simulink model "robotarm"  (R2018b)
settings: Solver=FixedStepAuto  StartTime=0.0  StopTime=20  RelTol=1e-3  AbsTol=1e-6
undefined symbols (not defined in the file or in its folder): options
libraries: neural x132, simulink x2
(part 2 of 6)

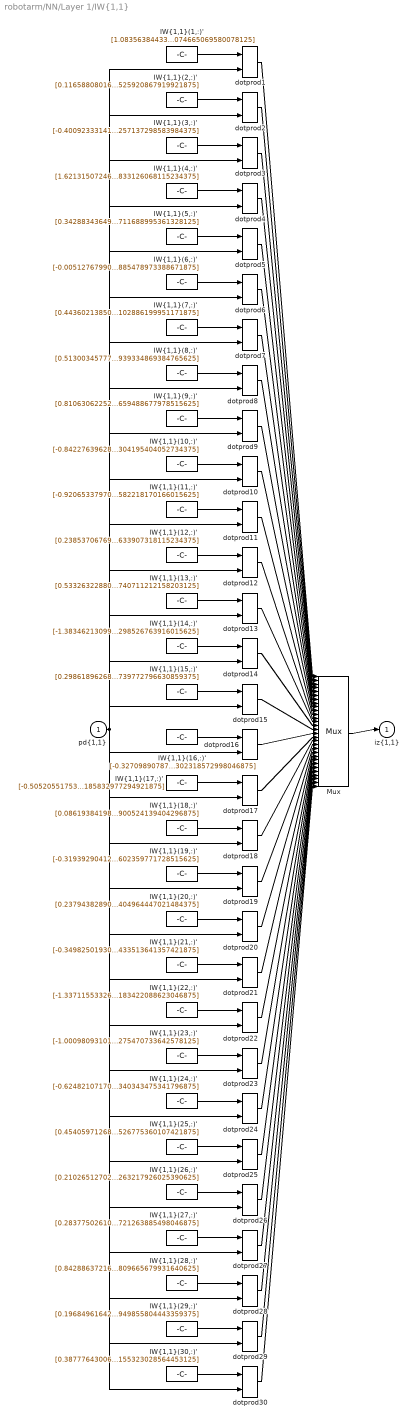
== system robotarm/NN/Layer 1/IW{1,1} ==
  "pd{1,1}" : Inport  PortDimensions=10
      mask Display: e = 0.06;c1 = [120 230 180]/255;c2 = ([120 230 180]+0)/(256+128);c3 = ([120 230 180]+128)/(256+128);patch([0 1 1 0],[0 0 1 1],c1);patch([0 1 1 1-e 1-e 0+e],[0 0 1 1-e 0+e 0+e],c2);patch([0 0 1 1-e 0+e 0+e],[0 1 1 1-e 1-e 0+e],c3);plot([0 1 1 0 0],[0 0 1 1 0]);
  "IW{1,1}(1,:)'" : Constant  Value=[1.083563844330424075224073021672666072845458984375;-0.419524106915114824989387898312998004257678985595703125;-0.94157120591915599572274686579476110637187957763671875;-0.01379674963687171039550261042450074455700814723968505859375;-0.58471965145644977379646434201276861131191253662109375;-0.280368088171196128133288993922178633511066436767578125;-0.31976801179407854380798426063847728073596954345703125;-0.52267253415010628270209736001561395823955535888671875;0.478910020528330815370310347134363837540149688720703125;0.1519211665722064730221774198071216233074665069580078125]
      mask Display: e = 0.06;c1 = [120 150 230]/255;c2 = ([120 150 230]+0)/383;c3 = ([120 150 230]+128)/383;patch([0 1 1 0],[0 0 1 1],c1);patch([0 1 1 1-e 1-e 0+e],[0 0 1 1-e 0+e 0+e],c2);patch([0 0 1 1-e 0+e 0+e],[0 1 1 1-e 1-e 0+e],c3);plot([0 1 1 0 0],[0 0 1 1 0]);disp('Weights');
  "IW{1,1}(10,:)'" : Constant  Value=[-0.842276396285047912471100062248297035694122314453125;-0.079177212965602150607224984923959709703922271728515625;0.61201067859849611618727749373647384345531463623046875;0.10430192382772003611979272363896598108112812042236328125;1.41024421573007874286531659890897572040557861328125;0.248495048171829047145564572929288260638713836669921875;-0.75706957483083592297390396197442896664142608642578125;0.472846624969997464393856034803320653736591339111328125;0.95744612924704741718784362092264927923679351806640625;1.4195525983288257432235468513681553304195404052734375]
      mask Display: e = 0.06;c1 = [120 150 230]/255;c2 = ([120 150 230]+0)/383;c3 = ([120 150 230]+128)/383;patch([0 1 1 0],[0 0 1 1],c1);patch([0 1 1 1-e 1-e 0+e],[0 0 1 1-e 0+e 0+e],c2);patch([0 0 1 1-e 0+e 0+e],[0 1 1 1-e 1-e 0+e],c3);plot([0 1 1 0 0],[0 0 1 1 0]);disp('Weights');
  "IW{1,1}(11,:)'" : Constant  Value=[-0.9206533797031231092233838353422470390796661376953125;1.000433613079543260226955680991522967815399169921875;-0.78174772750853949165872336379834450781345367431640625;0.9377401953158825964607103742309845983982086181640625;0.615533911757225826733019857783801853656768798828125;-1.301904266155556211259636256727389991283416748046875;-0.1439549990255313272058401707909069955348968505859375;-0.260988644890574217338752305295201949775218963623046875;-1.579813373534317832991291652433574199676513671875;0.3635611814509245309778862065286375582218170166015625]
      mask Display: e = 0.06;c1 = [120 150 230]/255;c2 = ([120 150 230]+0)/383;c3 = ([120 150 230]+128)/383;patch([0 1 1 0],[0 0 1 1],c1);patch([0 1 1 1-e 1-e 0+e],[0 0 1 1-e 0+e 0+e],c2);patch([0 0 1 1-e 0+e 0+e],[0 1 1 1-e 1-e 0+e],c3);plot([0 1 1 0 0],[0 0 1 1 0]);disp('Weights');
  "IW{1,1}(12,:)'" : Constant  Value=[0.2385370676987361993059977294251439161598682403564453125;-1.1182755603052239035122283894452266395092010498046875;0.30571718445612827697033253571134991943836212158203125;-0.12377321056275387978207191963520017452538013458251953125;-0.1540453467788618635569974912868929095566272735595703125;2.74495700415689203310876109753735363483428955078125;-2.15817502845816111545218518585897982120513916015625;0.12258293831009491048344983710194355808198451995849609375;0.435643584250738624685794775359681807458400726318359375;1.0191367826085675485359161029919050633907318115234375]
      mask Display: e = 0.06;c1 = [120 150 230]/255;c2 = ([120 150 230]+0)/383;c3 = ([120 150 230]+128)/383;patch([0 1 1 0],[0 0 1 1],c1);patch([0 1 1 1-e 1-e 0+e],[0 0 1 1-e 0+e 0+e],c2);patch([0 0 1 1-e 0+e 0+e],[0 1 1 1-e 1-e 0+e],c3);plot([0 1 1 0 0],[0 0 1 1 0]);disp('Weights');
  "IW{1,1}(13,:)'" : Constant  Value=[0.5332632288002676634874887895421124994754791259765625;-1.120563788042803654576573535450734198093414306640625;0.5760296974781053958025722749880515038967132568359375;0.1414568545696771317832229897248907946050167083740234375;-0.18376461551108647096697268352727405726909637451171875;0.748993908272824970850933823385275900363922119140625;-0.7624731059042806347036957959062419831752777099609375;0.1976752722123650551910856165704899467527866363525390625;0.07210207626949634296398272681472008116543292999267578125;0.5850282661990899857329395672422833740711212158203125]
      mask Display: e = 0.06;c1 = [120 150 230]/255;c2 = ([120 150 230]+0)/383;c3 = ([120 150 230]+128)/383;patch([0 1 1 0],[0 0 1 1],c1);patch([0 1 1 1-e 1-e 0+e],[0 0 1 1-e 0+e 0+e],c2);patch([0 0 1 1-e 0+e 0+e],[0 1 1 1-e 1-e 0+e],c3);plot([0 1 1 0 0],[0 0 1 1 0]);disp('Weights');
  "IW{1,1}(14,:)'" : Constant  Value=[-1.38346213099752279873655425035394728183746337890625;-0.6694901615044808185217561913304962217807769775390625;1.0052672642915541079133845414617098867893218994140625;-0.60839844430044476286667531894636340439319610595703125;1.978610543822657330537140296655707061290740966796875;0.08347416261820701788298748624583822675049304962158203125;-0.3532798783452408830640933956601656973361968994140625;-0.1049561498162090433794446653337217867374420166015625;-1.7363611870133974779406571542494930326938629150390625;0.2235057134043753335195248155287117697298526763916015625]
      mask Display: e = 0.06;c1 = [120 150 230]/255;c2 = ([120 150 230]+0)/383;c3 = ([120 150 230]+128)/383;patch([0 1 1 0],[0 0 1 1],c1);patch([0 1 1 1-e 1-e 0+e],[0 0 1 1-e 0+e 0+e],c2);patch([0 0 1 1-e 0+e 0+e],[0 1 1 1-e 1-e 0+e],c3);plot([0 1 1 0 0],[0 0 1 1 0]);disp('Weights');
  "IW{1,1}(15,:)'" : Constant  Value=[0.298618962681280020188268053971114568412303924560546875;-0.2574920415391714900721353842527605593204498291015625;0.286644932574378119571889556027599610388278961181640625;0.41670493839011901737734433481818996369838714599609375;0.9123539281340473650061539956368505954742431640625;-0.10092359044869168849256624298504902981221675872802734375;-1.363679620942679804329600301571190357208251953125;0.87390030526096407204050819927942939102649688720703125;0.1456549714138599682655694778077304363250732421875;0.58839728054712236993140095364651642739772796630859375]
      mask Display: e = 0.06;c1 = [120 150 230]/255;c2 = ([120 150 230]+0)/383;c3 = ([120 150 230]+128)/383;patch([0 1 1 0],[0 0 1 1],c1);patch([0 1 1 1-e 1-e 0+e],[0 0 1 1-e 0+e 0+e],c2);patch([0 0 1 1-e 0+e 0+e],[0 1 1 1-e 1-e 0+e],c3);plot([0 1 1 0 0],[0 0 1 1 0]);disp('Weights');
  "IW{1,1}(16,:)'" : Constant  Value=[-0.32709890787855167015862889456911943852901458740234375;-0.34977860185296594242032597321667708456516265869140625;0.159350112944072697107600333765731193125247955322265625;-0.4776914513121521821403803187422454357147216796875;0.28649800858607876730133057208149693906307220458984375;-1.6701621394718044744109874955029226839542388916015625;0.45311651717334289202199215651489794254302978515625;0.2452372552807220162929269235974061302840709686279296875;0.307275738364648998146577696388703770935535430908203125;-0.1802985558186971370986384499701671302318572998046875]
      mask Display: e = 0.06;c1 = [120 150 230]/255;c2 = ([120 150 230]+0)/383;c3 = ([120 150 230]+128)/383;patch([0 1 1 0],[0 0 1 1],c1);patch([0 1 1 1-e 1-e 0+e],[0 0 1 1-e 0+e 0+e],c2);patch([0 0 1 1-e 0+e 0+e],[0 1 1 1-e 1-e 0+e],c3);plot([0 1 1 0 0],[0 0 1 1 0]);disp('Weights');
  "IW{1,1}(17,:)'" : Constant  Value=[-0.505205517537357540192033411585725843906402587890625;0.73699201635039190971809830443817190825939178466796875;-0.91272025444561177831559461992583237588405609130859375;0.51464316420065514545711948812822811305522918701171875;-0.45956584150917467734842603022116236388683319091796875;0.266953627996282805145966676718671806156635284423828125;0.87997329801952528516295615190756507217884063720703125;0.56265541151544551379259928580722771584987640380859375;-0.81391511536075011878921259267372079193592071533203125;-0.17677379478027155368380363142932765185832977294921875]
      mask Display: e = 0.06;c1 = [120 150 230]/255;c2 = ([120 150 230]+0)/383;c3 = ([120 150 230]+128)/383;patch([0 1 1 0],[0 0 1 1],c1);patch([0 1 1 1-e 1-e 0+e],[0 0 1 1-e 0+e 0+e],c2);patch([0 0 1 1-e 0+e 0+e],[0 1 1 1-e 1-e 0+e],c3);plot([0 1 1 0 0],[0 0 1 1 0]);disp('Weights');
  "IW{1,1}(18,:)'" : Constant  Value=[0.08619384198746320169259860222155111841857433319091796875;0.229415038738241872096068618702702224254608154296875;0.422334408883638878773325586735154502093791961669921875;-0.0463857197077117422434611171411233954131603240966796875;-1.9378071193737458344230617512948811054229736328125;1.1617657080125656232638675646740011870861053466796875;0.72620292320079793402243240052484907209873199462890625;-0.266184247267512497092667445031111128628253936767578125;0.3750431508699769711512317371671088039875030517578125;0.12292905171981620415788682976199197582900524139404296875]
      mask Display: e = 0.06;c1 = [120 150 230]/255;c2 = ([120 150 230]+0)/383;c3 = ([120 150 230]+128)/383;patch([0 1 1 0],[0 0 1 1],c1);patch([0 1 1 1-e 1-e 0+e],[0 0 1 1-e 0+e 0+e],c2);patch([0 0 1 1-e 0+e 0+e],[0 1 1 1-e 1-e 0+e],c3);plot([0 1 1 0 0],[0 0 1 1 0]);disp('Weights');
  "IW{1,1}(19,:)'" : Constant  Value=[-0.319392904125261722914075335211236961185932159423828125;-1.11920722841916475687185084098018705844879150390625;1.2814339763144142469997177613549865782260894775390625;0.294714759578355245395187012036330997943878173828125;-0.127324947638250696169137654578662477433681488037109375;0.2780099290666580014175224278005771338939666748046875;-0.461406912688261894306407384647172875702381134033203125;0.946512221892773286668898435891605913639068603515625;-0.52604333433637762151846573033253662288188934326171875;1.12250699959288713358773748041130602359771728515625]
      mask Display: e = 0.06;c1 = [120 150 230]/255;c2 = ([120 150 230]+0)/383;c3 = ([120 150 230]+128)/383;patch([0 1 1 0],[0 0 1 1],c1);patch([0 1 1 1-e 1-e 0+e],[0 0 1 1-e 0+e 0+e],c2);patch([0 0 1 1-e 0+e 0+e],[0 1 1 1-e 1-e 0+e],c3);plot([0 1 1 0 0],[0 0 1 1 0]);disp('Weights');
  "IW{1,1}(2,:)'" : Constant  Value=[0.1165880801637612373955477096387767232954502105712890625;0.51480391570709194137833719651098363101482391357421875;0.85599582684588437775374814009410329163074493408203125;0.127689799126927516770280135460780002176761627197265625;-0.69251284680256031123235516133718192577362060546875;-0.77324080525538019248443788455915637314319610595703125;0.98812601958098100762839521848945878446102142333984375;-0.51915044520887076995308007099083624780178070068359375;0.35895177238562181454284427672973833978176116943359375;0.151165569358457652082705635621096007525920867919921875]
      mask Display: e = 0.06;c1 = [120 150 230]/255;c2 = ([120 150 230]+0)/383;c3 = ([120 150 230]+128)/383;patch([0 1 1 0],[0 0 1 1],c1);patch([0 1 1 1-e 1-e 0+e],[0 0 1 1-e 0+e 0+e],c2);patch([0 0 1 1-e 0+e 0+e],[0 1 1 1-e 1-e 0+e],c3);plot([0 1 1 0 0],[0 0 1 1 0]);disp('Weights');
  "IW{1,1}(20,:)'" : Constant  Value=[0.2379438289011180096554909368933294899761676788330078125;-1.3301846095986420426271479300339706242084503173828125;0.77044336265387458606568316099583171308040618896484375;-0.09547680704926130024201569312936044298112392425537109375;-2.715018010987653607202219063765369355678558349609375;2.072335550560776340489610447548329830169677734375;0.057260612174695142695401983701231074519455432891845703125;0.29725043610325474485733820984023623168468475341796875;-0.79005114949337118535055424217716790735721588134765625;-0.1293487886033327372015122591619729064404964447021484375]
      mask Display: e = 0.06;c1 = [120 150 230]/255;c2 = ([120 150 230]+0)/383;c3 = ([120 150 230]+128)/383;patch([0 1 1 0],[0 0 1 1],c1);patch([0 1 1 1-e 1-e 0+e],[0 0 1 1-e 0+e 0+e],c2);patch([0 0 1 1-e 0+e 0+e],[0 1 1 1-e 1-e 0+e],c3);plot([0 1 1 0 0],[0 0 1 1 0]);disp('Weights');
  "IW{1,1}(21,:)'" : Constant  Value=[-0.34982501930182452465345477321534417569637298583984375;0.451454660502078664041647471094620414078235626220703125;0.0176372183039427317396974359553496469743549823760986328125;0.5639563704868508775547297773300670087337493896484375;-0.61754695379530299970127771302941255271434783935546875;-1.1011264936744520337441599622252397239208221435546875;1.430952231708778388252767399535514414310455322265625;0.62703809529327825256217465721420012414455413818359375;0.89493822370913578279072453369735740125179290771484375;0.7420538838895331945622046987409703433513641357421875]
      mask Display: e = 0.06;c1 = [120 150 230]/255;c2 = ([120 150 230]+0)/383;c3 = ([120 150 230]+128)/383;patch([0 1 1 0],[0 0 1 1],c1);patch([0 1 1 1-e 1-e 0+e],[0 0 1 1-e 0+e 0+e],c2);patch([0 0 1 1-e 0+e 0+e],[0 1 1 1-e 1-e 0+e],c3);plot([0 1 1 0 0],[0 0 1 1 0]);disp('Weights');
  "IW{1,1}(22,:)'" : Constant  Value=[-1.3371155332655286773757552509778179228305816650390625;1.647611385498908731506162439472973346710205078125;0.7218372909033783368926151524647139012813568115234375;0.61517446653261964595316158010973595082759857177734375;0.4436209136289634979988250051974318921566009521484375;-0.618411794607119258415650620008818805217742919921875;0.03981089168389299881578580198038253001868724822998046875;0.204423240271942752155354128262843005359172821044921875;1.4694870831249475795488024232327006757259368896484375;0.34253618015753939385348303403588943183422088623046875]
      mask Display: e = 0.06;c1 = [120 150 230]/255;c2 = ([120 150 230]+0)/383;c3 = ([120 150 230]+128)/383;patch([0 1 1 0],[0 0 1 1],c1);patch([0 1 1 1-e 1-e 0+e],[0 0 1 1-e 0+e 0+e],c2);patch([0 0 1 1-e 0+e 0+e],[0 1 1 1-e 1-e 0+e],c3);plot([0 1 1 0 0],[0 0 1 1 0]);disp('Weights');
  "IW{1,1}(23,:)'" : Constant  Value=[-1.000980931013797370354723170748911798000335693359375;0.478833175182671821890068031279952265322208404541015625;0.94978064588756883068754177656956017017364501953125;1.1443594633221680911816520165302790701389312744140625;-0.11379400009978284102896139984295587055385112762451171875;0.74083642701004481789794908763724379241466522216796875;1.2769530613015283027067425791756249964237213134765625;-0.625360364122677925280413546715863049030303955078125;0.771054043074430150994658106355927884578704833984375;0.00902667251292374635263104920568366651423275470733642578125]
      mask Display: e = 0.06;c1 = [120 150 230]/255;c2 = ([120 150 230]+0)/383;c3 = ([120 150 230]+128)/383;patch([0 1 1 0],[0 0 1 1],c1);patch([0 1 1 1-e 1-e 0+e],[0 0 1 1-e 0+e 0+e],c2);patch([0 0 1 1-e 0+e 0+e],[0 1 1 1-e 1-e 0+e],c3);plot([0 1 1 0 0],[0 0 1 1 0]);disp('Weights');
  "IW{1,1}(24,:)'" : Constant  Value=[-0.6248210717015967308185508954920805990695953369140625;0.08457395706912758381879058333652210421860218048095703125;0.51798080722533257347350854615797288715839385986328125;-0.2401174058161140434375369068220607005059719085693359375;0.268766942934225816497217920186812989413738250732421875;-1.0091454203326735150625381720601581037044525146484375;0.3587305078967546467794136333395726978778839111328125;0.6470235736711653640185204494628123939037322998046875;-0.7765010235893623491421067228657193481922149658203125;-0.336555415051090267564148916790145449340343475341796875]
      mask Display: e = 0.06;c1 = [120 150 230]/255;c2 = ([120 150 230]+0)/383;c3 = ([120 150 230]+128)/383;patch([0 1 1 0],[0 0 1 1],c1);patch([0 1 1 1-e 1-e 0+e],[0 0 1 1-e 0+e 0+e],c2);patch([0 0 1 1-e 0+e 0+e],[0 1 1 1-e 1-e 0+e],c3);plot([0 1 1 0 0],[0 0 1 1 0]);disp('Weights');
  "IW{1,1}(25,:)'" : Constant  Value=[0.454059712686064653741624397298437543213367462158203125;-1.3517731457203157052759934231289662420749664306640625;0.1376707745836474316991626665185322053730487823486328125;-0.117666794937914265251066581186023540794849395751953125;0.1560771799800420300829983943913248367607593536376953125;-1.0269078294976130560911542488611303269863128662109375;-0.0027601815689167748073262753649714795756153762340545654296875;0.72699730352820690626458599581383168697357177734375;0.283288442579868571247203590246499516069889068603515625;1.308014024318274959313157523865811526775360107421875]
      mask Display: e = 0.06;c1 = [120 150 230]/255;c2 = ([120 150 230]+0)/383;c3 = ([120 150 230]+128)/383;patch([0 1 1 0],[0 0 1 1],c1);patch([0 1 1 1-e 1-e 0+e],[0 0 1 1-e 0+e 0+e],c2);patch([0 0 1 1-e 0+e 0+e],[0 1 1 1-e 1-e 0+e],c3);plot([0 1 1 0 0],[0 0 1 1 0]);disp('Weights');
  "IW{1,1}(26,:)'" : Constant  Value=[0.210265127027331522047148837373242713510990142822265625;-0.48581145213011378558576325303874909877777099609375;-0.123258874216255642775053047444089315831661224365234375;1.3525906749941525308855716502876020967960357666015625;-0.67024790288814617422730179896461777389049530029296875;-0.100694977273113772664459020234062336385250091552734375;-0.472021084205861474192289506390807218849658966064453125;-0.12293932717995796621845983054299722425639629364013671875;1.4301368055528242972940233812551014125347137451171875;-0.5388690494755474791332972017698921263217926025390625]
      mask Display: e = 0.06;c1 = [120 150 230]/255;c2 = ([120 150 230]+0)/383;c3 = ([120 150 230]+128)/383;patch([0 1 1 0],[0 0 1 1],c1);patch([0 1 1 1-e 1-e 0+e],[0 0 1 1-e 0+e 0+e],c2);patch([0 0 1 1-e 0+e 0+e],[0 1 1 1-e 1-e 0+e],c3);plot([0 1 1 0 0],[0 0 1 1 0]);disp('Weights');
  "IW{1,1}(27,:)'" : Constant  Value=[0.283775026102151828322206483790068887174129486083984375;-1.009030341954201492882248203386552631855010986328125;0.487583465416730976738080016730236820876598358154296875;-0.18846379806061719364151940681040287017822265625;-0.058983956930411328423158323630559607408940792083740234375;1.64386081481786394675737028592266142368316650390625;-0.40826383464646998078251272090710699558258056640625;0.033231970936722636522642204681687871925532817840576171875;-0.85776196289379547099684941713348962366580963134765625;-0.510846364679220510396362442406825721263885498046875]
      mask Display: e = 0.06;c1 = [120 150 230]/255;c2 = ([120 150 230]+0)/383;c3 = ([120 150 230]+128)/383;patch([0 1 1 0],[0 0 1 1],c1);patch([0 1 1 1-e 1-e 0+e],[0 0 1 1-e 0+e 0+e],c2);patch([0 0 1 1-e 0+e 0+e],[0 1 1 1-e 1-e 0+e],c3);plot([0 1 1 0 0],[0 0 1 1 0]);disp('Weights');
  "IW{1,1}(28,:)'" : Constant  Value=[0.84288637216753314884698511377791874110698699951171875;-0.413855342383396107575066480421810410916805267333984375;0.4049198819575854368935097227222286164760589599609375;-0.68308376935264780716039467733935452997684478759765625;-0.30854675245235763103579529342823661863803863525390625;-0.8917618698073483951560547211556695401668548583984375;-0.0897240545776623876772504218024550937116146087646484375;0.29103135192875873027418265337473712861537933349609375;0.5568927271626560315809228995931334793567657470703125;1.0573139604906318655963559649535454809665679931640625]
      mask Display: e = 0.06;c1 = [120 150 230]/255;c2 = ([120 150 230]+0)/383;c3 = ([120 150 230]+128)/383;patch([0 1 1 0],[0 0 1 1],c1);patch([0 1 1 1-e 1-e 0+e],[0 0 1 1-e 0+e 0+e],c2);patch([0 0 1 1-e 0+e 0+e],[0 1 1 1-e 1-e 0+e],c3);plot([0 1 1 0 0],[0 0 1 1 0]);disp('Weights');
  "IW{1,1}(29,:)'" : Constant  Value=[0.1968496164217669319729253629702725447714328765869140625;-1.4750248961380225676265354195493273437023162841796875;-0.0731711881804112673766127272756421007215976715087890625;-0.15866772515695803935642516080406494438648223876953125;0.25971984401405634468318339713732711970806121826171875;0.494830116170369038730569855033536441624164581298828125;-1.1275228062812632234823695398517884314060211181640625;0.387494119223098676396688233580789528787136077880859375;-0.260836540485615275830610926277586258947849273681640625;0.850286234828498521665096632204949855804443359375]
      mask Display: e = 0.06;c1 = [120 150 230]/255;c2 = ([120 150 230]+0)/383;c3 = ([120 150 230]+128)/383;patch([0 1 1 0],[0 0 1 1],c1);patch([0 1 1 1-e 1-e 0+e],[0 0 1 1-e 0+e 0+e],c2);patch([0 0 1 1-e 0+e 0+e],[0 1 1 1-e 1-e 0+e],c3);plot([0 1 1 0 0],[0 0 1 1 0]);disp('Weights');
  "IW{1,1}(3,:)'" : Constant  Value=[-0.400923331416590145170886216874350793659687042236328125;-0.1476879098288665925764462372171692550182342529296875;0.13125453123017549739159903765539638698101043701171875;0.04264655243906863291147857353280414827167987823486328125;0.72609917272249735464839659471181221306324005126953125;-1.075400786488810211949385120533406734466552734375;-0.0879519664267141842994846001602127216756343841552734375;0.11714601634093980975226401142208487726747989654541015625;1.68484348980962561626029128092341125011444091796875;0.145654699934613718337317322948365472257137298583984375]
      mask Display: e = 0.06;c1 = [120 150 230]/255;c2 = ([120 150 230]+0)/383;c3 = ([120 150 230]+128)/383;patch([0 1 1 0],[0 0 1 1],c1);patch([0 1 1 1-e 1-e 0+e],[0 0 1 1-e 0+e 0+e],c2);patch([0 0 1 1-e 0+e 0+e],[0 1 1 1-e 1-e 0+e],c3);plot([0 1 1 0 0],[0 0 1 1 0]);disp('Weights');
  "IW{1,1}(30,:)'" : Constant  Value=[0.387776430068318134214422343575279228389263153076171875;-0.0647149855580241017971587780266418121755123138427734375;-0.1699837310918328459052872858592309057712554931640625;-0.80075379385953004973686120138154365122318267822265625;-1.2626851263460927565773772585089318454265594482421875;0.011167974204610929545022912634522072039544582366943359375;-0.5182507885322260587912523988052271306514739990234375;1.2029977843526695746589894042699597775936126708984375;0.75153166640015722776979600894264876842498779296875;-0.50937516538142280086987057075020857155323028564453125]
      mask Display: e = 0.06;c1 = [120 150 230]/255;c2 = ([120 150 230]+0)/383;c3 = ([120 150 230]+128)/383;patch([0 1 1 0],[0 0 1 1],c1);patch([0 1 1 1-e 1-e 0+e],[0 0 1 1-e 0+e 0+e],c2);patch([0 0 1 1-e 0+e 0+e],[0 1 1 1-e 1-e 0+e],c3);plot([0 1 1 0 0],[0 0 1 1 0]);disp('Weights');
  "IW{1,1}(4,:)'" : Constant  Value=[1.6213150724644496136761517846025526523590087890625;-1.39679987700754093538080269354395568370819091796875;-0.332220191857820756897723413203493691980838775634765625;0.53809858749224026563950928903068415820598602294921875;0.63296520357793617517216944179381243884563446044921875;-0.59547763359107486191845737266703508794307708740234375;-0.1773979392923067111009771679164259694516658782958984375;-0.0418584878074302613182311461059725843369960784912109375;0.65839587112526920531507812484051100909709930419921875;-0.025669197067267078560259818686972721479833126068115234375]
      mask Display: e = 0.06;c1 = [120 150 230]/255;c2 = ([120 150 230]+0)/383;c3 = ([120 150 230]+128)/383;patch([0 1 1 0],[0 0 1 1],c1);patch([0 1 1 1-e 1-e 0+e],[0 0 1 1-e 0+e 0+e],c2);patch([0 0 1 1-e 0+e 0+e],[0 1 1 1-e 1-e 0+e],c3);plot([0 1 1 0 0],[0 0 1 1 0]);disp('Weights');
  "IW{1,1}(5,:)'" : Constant  Value=[0.342883436499595017910024807861191220581531524658203125;-1.041725722576007484576621209271252155303955078125;1.0054712358771265012791218396159820258617401123046875;-0.1703917873305470787048676584163331426680088043212890625;-1.1231709362679265229445491058868356049060821533203125;-0.8999364133153096023676198456087149679660797119140625;1.001279779505041656051389509229920804500579833984375;0.520364571732873759657422851887531578540802001953125;-0.90843751779553638669995052623562514781951904296875;-0.5052734573743038470894362035323865711688995361328125]
      mask Display: e = 0.06;c1 = [120 150 230]/255;c2 = ([120 150 230]+0)/383;c3 = ([120 150 230]+128)/383;patch([0 1 1 0],[0 0 1 1],c1);patch([0 1 1 1-e 1-e 0+e],[0 0 1 1-e 0+e 0+e],c2);patch([0 0 1 1-e 0+e 0+e],[0 1 1 1-e 1-e 0+e],c3);plot([0 1 1 0 0],[0 0 1 1 0]);disp('Weights');
  "IW{1,1}(6,:)'" : Constant  Value=[-0.005127679904386222599355082962802043766714632511138916015625;0.0253848319082346229880187138405744917690753936767578125;-0.62515248241674992168981361828627996146678924560546875;-0.1283637197299608845302287818412878550589084625244140625;-1.9671894012805564155854654018185101449489593505859375;1.0825371931026896987759755575098097324371337890625;0.035051283613600346666938634143662056885659694671630859375;0.749323223085553546951587122748605906963348388671875;-0.96344846650526727582786179482354782521724700927734375;0.357009315324879394903945240002940408885478973388671875]
      mask Display: e = 0.06;c1 = [120 150 230]/255;c2 = ([120 150 230]+0)/383;c3 = ([120 150 230]+128)/383;patch([0 1 1 0],[0 0 1 1],c1);patch([0 1 1 1-e 1-e 0+e],[0 0 1 1-e 0+e 0+e],c2);patch([0 0 1 1-e 0+e 0+e],[0 1 1 1-e 1-e 0+e],c3);plot([0 1 1 0 0],[0 0 1 1 0]);disp('Weights');
  "IW{1,1}(7,:)'" : Constant  Value=[0.443602138500584108893320944844163022935390472412109375;0.5897042425490841566215749480761587619781494140625;-0.07776107471227244882783224966260604560375213623046875;0.73813404077385735835292734918766655027866363525390625;-1.0677992091214718595182375793228857219219207763671875;1.0308052764952078117488554198644123971462249755859375;0.346772813933108547956862821592949330806732177734375;-0.15978460419619111565481262005050666630268096923828125;-0.577740532505497839110830682329833507537841796875;-1.103881593575507746862740532378666102886199951171875]
      mask Display: e = 0.06;c1 = [120 150 230]/255;c2 = ([120 150 230]+0)/383;c3 = ([120 150 230]+128)/383;patch([0 1 1 0],[0 0 1 1],c1);patch([0 1 1 1-e 1-e 0+e],[0 0 1 1-e 0+e 0+e],c2);patch([0 0 1 1-e 0+e 0+e],[0 1 1 1-e 1-e 0+e],c3);plot([0 1 1 0 0],[0 0 1 1 0]);disp('Weights');
  "IW{1,1}(8,:)'" : Constant  Value=[0.5130034577743221024803688123938627541065216064453125;-1.36132327419380683153349309577606618404388427734375;-0.184786816108494955646079915823065675795078277587890625;0.57684124394947866587557427919819019734859466552734375;-0.80847892494082407299771375619457103312015533447265625;0.13647065469038854867989130070782266557216644287109375;-0.69725806686932312317139803781174123287200927734375;-0.49791543974283591911245139272068627178668975830078125;0.5568004775091164315625746894511394202709197998046875;-0.56237914196716209946913522799150086939334869384765625]
      mask Display: e = 0.06;c1 = [120 150 230]/255;c2 = ([120 150 230]+0)/383;c3 = ([120 150 230]+128)/383;patch([0 1 1 0],[0 0 1 1],c1);patch([0 1 1 1-e 1-e 0+e],[0 0 1 1-e 0+e 0+e],c2);patch([0 0 1 1-e 0+e 0+e],[0 1 1 1-e 1-e 0+e],c3);plot([0 1 1 0 0],[0 0 1 1 0]);disp('Weights');
  "IW{1,1}(9,:)'" : Constant  Value=[0.810630622529874056425569506245665252208709716796875;0.13529562971586173159010968447546474635601043701171875;-0.08447588975580629100381457874391344375908374786376953125;0.173504432054140289576338318511261604726314544677734375;-1.2880709604838729287479281993000768125057220458984375;-1.4583641511193936590728981173015199601650238037109375;2.08180199668271370683214627206325531005859375;0.6387697649847867698014169945963658392429351806640625;-0.39397763097241222940425586784840561449527740478515625;-0.05706823956178132262184732326204539276659488677978515625]
      mask Display: e = 0.06;c1 = [120 150 230]/255;c2 = ([120 150 230]+0)/383;c3 = ([120 150 230]+128)/383;patch([0 1 1 0],[0 0 1 1],c1);patch([0 1 1 1-e 1-e 0+e],[0 0 1 1-e 0+e 0+e],c2);patch([0 0 1 1-e 0+e 0+e],[0 1 1 1-e 1-e 0+e],c3);plot([0 1 1 0 0],[0 0 1 1 0]);disp('Weights');
  Mux : Mux  Inputs=30
      mask Display: e = 0.06;c1 = [120 150 230]/255;c2 = ([120 150 230]+0)/383;c3 = ([120 150 230]+128)/383;patch([0 1 1 0],[0 0 1 1],c1);patch([0 1 1 1-e 1-e 0+e],[0 0 1 1-e 0+e 0+e],c2);patch([0 0 1 1-e 0+e 0+e],[0 1 1 1-e 1-e 0+e],c3);plot([0 1 1 0 0],[0 0 1 1 0]);disp('Mux');
  dotprod{1..30} (30 alike) : neural/Weight Functions/dotprod
  "iz{1,1}" : Outport
      mask Display: e = 0.06;c1 = [120 230 180]/255;c2 = ([120 230 180]+0)/(256+128);c3 = ([120 230 180]+128)/(256+128);patch([0 1 1 0],[0 0 1 1],c1);patch([0 1 1 1-e 1-e 0+e],[0 0 1 1-e 0+e 0+e],c2);patch([0 0 1 1-e 0+e 0+e],[0 1 1 1-e 1-e 0+e],c3);plot([0 1 1 0 0],[0 0 1 1 0]);
  wires:
  "IW{1,1}(1,:)'"/1 -> dotprod1/1
  "pd{1,1}"/1 -> dotprod1/2, dotprod2/2, dotprod3/2, dotprod4/2, dotprod5/2, dotprod6/2, dotprod7/2, dotprod8/2, dotprod9/2, dotprod10/2, dotprod11/2, dotprod12/2, dotprod13/2, dotprod14/2, dotprod15/2, dotprod16/2, dotprod17/2, dotprod18/2, dotprod19/2, dotprod20/2, dotprod21/2, dotprod22/2, dotprod23/2, dotprod24/2, dotprod25/2, dotprod26/2, dotprod27/2, dotprod28/2, dotprod29/2, dotprod30/2
  dotprod1/1 -> Mux/1
  "IW{1,1}(2,:)'"/1 -> dotprod2/1
  dotprod2/1 -> Mux/2
  "IW{1,1}(3,:)'"/1 -> dotprod3/1
  dotprod3/1 -> Mux/3
  "IW{1,1}(4,:)'"/1 -> dotprod4/1
  dotprod4/1 -> Mux/4
  "IW{1,1}(5,:)'"/1 -> dotprod5/1
  dotprod5/1 -> Mux/5
  "IW{1,1}(6,:)'"/1 -> dotprod6/1
  dotprod6/1 -> Mux/6
  "IW{1,1}(7,:)'"/1 -> dotprod7/1
  dotprod7/1 -> Mux/7
  "IW{1,1}(8,:)'"/1 -> dotprod8/1
  dotprod8/1 -> Mux/8
  "IW{1,1}(9,:)'"/1 -> dotprod9/1
  dotprod9/1 -> Mux/9
  "IW{1,1}(10,:)'"/1 -> dotprod10/1
  dotprod10/1 -> Mux/10
  "IW{1,1}(11,:)'"/1 -> dotprod11/1
  dotprod11/1 -> Mux/11
  "IW{1,1}(12,:)'"/1 -> dotprod12/1
  dotprod12/1 -> Mux/12
  "IW{1,1}(13,:)'"/1 -> dotprod13/1
  dotprod13/1 -> Mux/13
  "IW{1,1}(14,:)'"/1 -> dotprod14/1
  dotprod14/1 -> Mux/14
  "IW{1,1}(15,:)'"/1 -> dotprod15/1
  dotprod15/1 -> Mux/15
  "IW{1,1}(16,:)'"/1 -> dotprod16/1
  dotprod16/1 -> Mux/16
  "IW{1,1}(17,:)'"/1 -> dotprod17/1
  dotprod17/1 -> Mux/17
  "IW{1,1}(18,:)'"/1 -> dotprod18/1
  dotprod18/1 -> Mux/18
  "IW{1,1}(19,:)'"/1 -> dotprod19/1
  dotprod19/1 -> Mux/19
  "IW{1,1}(20,:)'"/1 -> dotprod20/1
  dotprod20/1 -> Mux/20
  "IW{1,1}(21,:)'"/1 -> dotprod21/1
  dotprod21/1 -> Mux/21
  "IW{1,1}(22,:)'"/1 -> dotprod22/1
  dotprod22/1 -> Mux/22
  "IW{1,1}(23,:)'"/1 -> dotprod23/1
  dotprod23/1 -> Mux/23
  "IW{1,1}(24,:)'"/1 -> dotprod24/1
  dotprod24/1 -> Mux/24
  "IW{1,1}(25,:)'"/1 -> dotprod25/1
  dotprod25/1 -> Mux/25
  "IW{1,1}(26,:)'"/1 -> dotprod26/1
  dotprod26/1 -> Mux/26
  "IW{1,1}(27,:)'"/1 -> dotprod27/1
  dotprod27/1 -> Mux/27
  "IW{1,1}(28,:)'"/1 -> dotprod28/1
  dotprod28/1 -> Mux/28
  "IW{1,1}(29,:)'"/1 -> dotprod29/1
  dotprod29/1 -> Mux/29
  "IW{1,1}(30,:)'"/1 -> dotprod30/1
  dotprod30/1 -> Mux/30
  Mux/1 -> "iz{1,1}"/1

== system robotarm/NN/Layer 2/Delays 1 ==
  "p{2}" : Inport  PortDimensions=30
      mask Display: e = 0.06;c1 = [120 230 180]/255;c2 = ([120 230 180]+0)/(256+128);c3 = ([120 230 180]+128)/(256+128);patch([0 1 1 0],[0 0 1 1],c1);patch([0 1 1 1-e 1-e 0+e],[0 0 1 1-e 0+e 0+e],c2);patch([0 0 1 1-e 0+e 0+e],[0 1 1 1-e 1-e 0+e],c3);plot([0 1 1 0 0],[0 0 1 1 0]);
  mux : Mux  Inputs=1
      mask Display: e = 0.06;c1 = [120 150 230]/255;c2 = ([120 150 230]+0)/383;c3 = ([120 150 230]+128)/383;patch([0 1 1 0],[0 0 1 1],c1);patch([0 1 1 1-e 1-e 0+e],[0 0 1 1-e 0+e 0+e],c2);patch([0 0 1 1-e 0+e 0+e],[0 1 1 1-e 1-e 0+e],c3);plot([0 1 1 0 0],[0 0 1 1 0]);disp('Mux')
  "pd{2,1}" : Outport
      mask Display: e = 0.06;c1 = [120 230 180]/255;c2 = ([120 230 180]+0)/(256+128);c3 = ([120 230 180]+128)/(256+128);patch([0 1 1 0],[0 0 1 1],c1);patch([0 1 1 1-e 1-e 0+e],[0 0 1 1-e 0+e 0+e],c2);patch([0 0 1 1-e 0+e 0+e],[0 1 1 1-e 1-e 0+e],c3);plot([0 1 1 0 0],[0 0 1 1 0]);
  wires:
  "p{2}"/1 -> mux/1
  mux/1 -> "pd{2,1}"/1
